simulink model "controlPosicion"  (R2020a)
settings: Solver=VariableStepAuto  StartTime=0.0  StopTime=10.0  RelTol=1e-3
libraries: roblocks x1
settings Model: Creator=Marcelo  LastModifiedBy=Marcelo

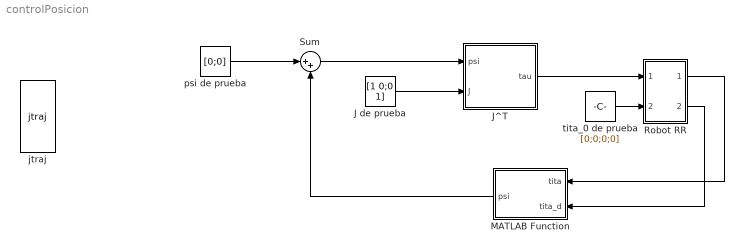
== system controlPosicion ==
  J de prueba : Constant  Value=[1 0;0 1]
  J^T : MATLAB Function  TreatAsAtomicUnit=on
  MATLAB Function : MATLAB Function  TreatAsAtomicUnit=on
  Robot RR : Subsystem
  Sum : Sum  Inputs=|++
  jtraj : roblocks/Toolbox/jtraj  q0=[1 -1]  qf=[1 1]  tmax=10  ts=0.02
  psi de prueba : Constant  Value=[0;0]
  tita_0 de prueba : Constant  Value=[0;0;0;0]
  wires:
  Sum/1 -> J^T/1(psi)
  J^T/1(tau) -> Robot RR/1(tau)
  Robot RR/1(tita) -> MATLAB Function/1(tita)
  Robot RR/2(tita_d) -> MATLAB Function/2(tita_d)
  MATLAB Function/1(psi) -> Sum/2
  psi de prueba/1 -> Sum/1
  tita_0 de prueba/1 -> Robot RR/2(tita_0)
  J de prueba/1 -> J^T/2(J)

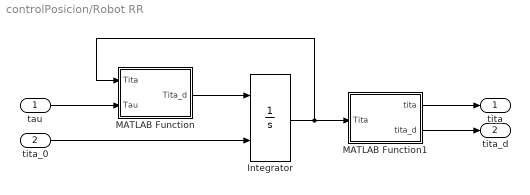
== system controlPosicion/Robot RR ==
  tau : Inport
  tita_0 : Inport  Port=2
  Integrator : Integrator  InitialConditionSource=external
  MATLAB Function : MATLAB Function  TreatAsAtomicUnit=on
  MATLAB Function1 : MATLAB Function  TreatAsAtomicUnit=on
  tita : Outport
  tita_d : Outport  Port=2
  wires:
  tau/1 -> MATLAB Function/2(Tau)
  MATLAB Function/1(Tita_d) -> Integrator/1
  tita_0/1 -> Integrator/2
  Integrator/1 -> MATLAB Function1/1(Tita), MATLAB Function/1(Tita)
  MATLAB Function1/1(tita) -> tita/1
  MATLAB Function1/2(tita_d) -> tita_d/1

== matlab function controlPosicion/J^T ==
  data: psi input; tau output; J input
function tau = fcn(psi,J)

tau = J'*psi;

== matlab function controlPosicion/Robot RR/MATLAB Function ==
  data: Tita input; Tita_d output; Tau input
function Tita_d = fcn(Tita,Tau)

titad1 = Tita(2);
titadd1 = Tau(1)+10*cos(Tita(1))-Tita(2);
titad2 = Tau(2);
titadd2 = 0;

Tita_d = [titad1;titadd1;titad2;titadd2];

== matlab function controlPosicion/Robot RR/MATLAB Function1 ==
  data: Tita input; tita output; tita_d output
function [tita,tita_d] = fcn(Tita)

tita = [Tita(1);Tita(3)];
tita_d = [Tita(2);Tita(4)];

== matlab function controlPosicion/MATLAB Function ==
  data: tita input; psi output; tita_d input
function psi = f(tita,tita_d)

psi1 = +10*cos(tita(1))-tita_d(1);
psi2 = -tita_d(2);

psi = [psi1;psi2];
